simulink model "Control_model_10DOF_fin"  (R2016b)
settings: Solver=FixedStepAuto  StartTime=0.0  StopTime=10  FixedStep=0.0001  RelTol=1e-3
InitFcn:
  | Initialisation_ctr_10DOF_fin
values from neighbouring files (symbols this model uses):
  COM_Parameters = [-lpelvis/2;r2;0]    [Initialisation_ctr_10DOF_fin.m]
  DH_Parameters = [hfoot 0 ... (first row only)    [Initialisation_ctr_10DOF_fin.m]
  dTrunk = trunklbd(3)    [Initialisation_ctr_10DOF_fin.m]
  dxFootSM = dxFoot    [Initialisation_ctr_10DOF_fin.m]
  dxTrunk = 0.1    [Initialisation_ctr_10DOF_fin.m]
  Foot_Parameters = [0;-(lFoot/2-lHeel);0]    [Initialisation_ctr_10DOF_fin.m]
  HAA2HEE = [0; 0; 0.001]    [Initialisation_ctr_10DOF_fin.m]
  HEE2HFE = 0.5*[0.2; 0; 0]    [Initialisation_ctr_10DOF_fin.m]
  height_vrp = CoM_position(1)    [Initialisation_ctr_10DOF_fin.m]
  hTrunk = trunklbd(1)    [Initialisation_ctr_10DOF_fin.m]
  initial_CoM_position = R*CoM_position    [Initialisation_ctr_10DOF_fin.m]
  initial_CoM_velocity = [0;0;0]    [Initialisation_ctr_10DOF_fin.m]
  initial_left_foot = [0;0;-stance_width/2]    [Initialisation_ctr_10DOF_fin.m]
  initial_right_foot = [0;0;stance_width/2]    [Initialisation_ctr_10DOF_fin.m]
  initial_RorL = 0    [Initialisation_ctr_10DOF_fin.m]
  jointsinitial = [9;-15;6;0;0;6;-15;9]/180*pi    [Initialisation_ctr_10DOF_fin.m]
  K_DCM = 4.3*[1 0 0 ... (first row only)    [Initialisation_ctr_10DOF_fin.m]
  kD_left = mbody*[0.95 0 0 0 ... (first row only)    [Initialisation_ctr_10DOF_fin.m]
  kD_right = mbody*[0.12 0 0 0 ... (first row only)    [Initialisation_ctr_10DOF_fin.m]
  kI_left = mbody*[35 0 0 0 ... (first row only)    [Initialisation_ctr_10DOF_fin.m]
  kI_right = mbody*[38.2 0 0 0 ... (first row only)    [Initialisation_ctr_10DOF_fin.m]
  kP_left = mbody*[75 0 0 0 ... (first row only)    [Initialisation_ctr_10DOF_fin.m]
  kP_right = mbody*[5.6 0 0 0 ... (first row only)    [Initialisation_ctr_10DOF_fin.m]
  Lenght = [lShank;lThigh]    [Initialisation_ctr_10DOF_fin.m]
  lFootSM = lFoot    [Initialisation_ctr_10DOF_fin.m]
  lpelvis = wPelvis    [Initialisation_ctr_10DOF_fin.m]
  mass = mbody    (= 60)    [Initialisation_ctr_10DOF_fin.m]
  Masses = [mThigh; mShank; mTrunk]    [Initialisation_ctr_10DOF_fin.m]
  nb_step = 4    [Initialisation_ctr_10DOF_fin.m]
  nb_step_pattern = 20    [Initialisation_ctr_10DOF_fin.m]
  Pelvis_Parameters = [-lpelvis/2;hTrunk/2;0]    [Initialisation_ctr_10DOF_fin.m]
  stance_width = lpelvis    [Initialisation_ctr_10DOF_fin.m]
  stride_lenght = 0.50    (= 0.5)    [Initialisation_ctr_10DOF_fin.m]
  T_DS = time_DS    (= 0.4)    [Initialisation_ctr_10DOF_fin.m]
  T_IT = time_DS    (= 0.4)    [Initialisation_ctr_10DOF_fin.m]
  T_SS = time_swing    (= 1.6)    [Initialisation_ctr_10DOF_fin.m]
  time_DS = (time_stance-time_swing)/2    (= 0.4)    [Initialisation_ctr_10DOF_fin.m]
  time_stance = 60/100*time_stride    (= 2.4)    [Initialisation_ctr_10DOF_fin.m]
  time_step = time_stride/2    (= 2)    [Initialisation_ctr_10DOF_fin.m]
  time_swing = 40/100*time_stride    (= 1.6)    [Initialisation_ctr_10DOF_fin.m]
  validity_angle = [-20*pi/180 20*pi/180 ... (first row only)    [Initialisation_ctr_10DOF_fin.m]
  wTrunk = trunklbd(2)    [Initialisation_ctr_10DOF_fin.m]
  x4CoM = CoM_position(1)-XR4(1)    [Initialisation_ctr_10DOF_fin.m]
undefined symbols (not defined in the file or in its folder): dsegment, hFoot, l, lFoot, omega0_x, omega0_z, rho, wPelvis, X, Xp_x, Xp_z, Y, Z
undefined symbols (not defined in the file): k_grf, lShankSM, lThighSM, mShank, mThigh
libraries: nesl_utility x247, sm_lib x215, dspindex x12, FootPlacementLibrary x8, dspsigops x4, dspswit3 x1
(part 12 of 18)

== system Control_model_10DOF_fin/Control/Single_Support/Left Swing // Right Stance/Left Swing leg control/Scope x2 ==
  Input : Inport
  Input1 : Inport  Port=2
  Demux : Demux
  Demux1 : Demux
  Scope{,1..3} (4 alike) : Scope  NumInputPorts=2
  wires:
  Input/1 -> Demux/1
  Demux/2 -> Scope1/1
  Demux/3 -> Scope2/1
  Demux/1 -> Scope3/1
  Input1/1 -> Demux1/1
  Demux1/1 -> Scope3/2
  Demux1/2 -> Scope1/2
  Demux1/3 -> Scope2/2
  Demux1/4 -> Scope/2
  Demux/4 -> Scope/1

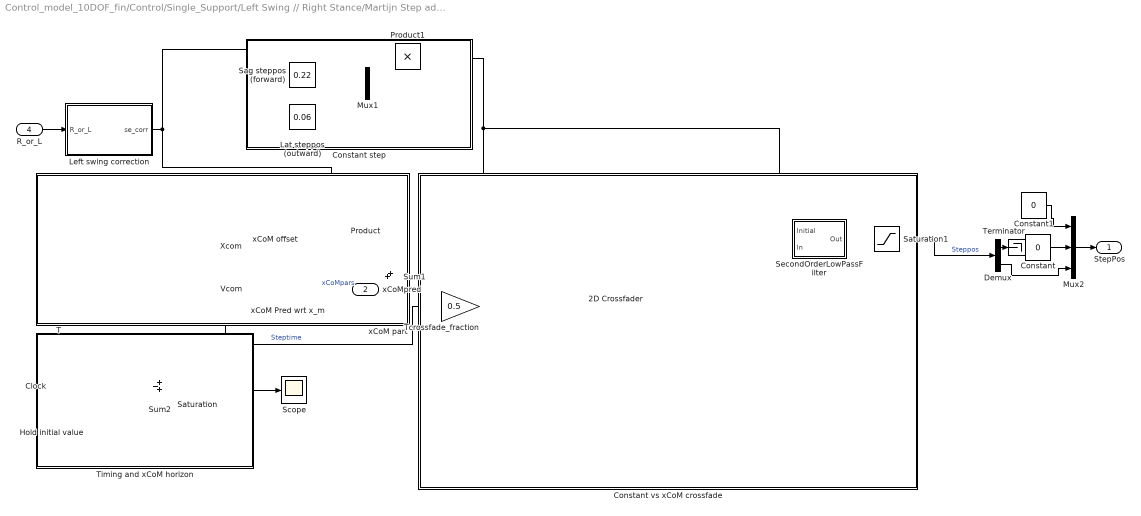
== system Control_model_10DOF_fin/Control/Single_Support/Left Swing // Right Stance/Martijn Step adjustement/xCoM pred ==
  T : Inport
  Xcom : Inport  Port=2
  Vcom : Inport  Port=3
  R_or_L : Inport  Port=4
  2D Crossfader : Subsystem
  Clock : Clock
  Constant : Constant  Value=0
  Constant step : Subsystem
  Constant vs xCoM crossfade : Subsystem
  Constant1 : Constant  Value=0
  Demux : Demux  Outputs=2
  Hold initial value : FootPlacementLibrary/Hold initial value  SystemSampleTime=-1
  Lat steppos (outward) : Constant  Value=0.06
  Left swing correction : Subsystem
  Mux1 : Mux  Inputs=2
  Mux2 : Mux  Inputs=3
  Product : Product
  Product1 : Product
  Sag steppos (forward) : Constant  Value=0.22
  Saturation : Saturate  UpperLimit=0.75  LowerLimit=0
  Saturation1 : Saturate  UpperLimit=[0.3 0.4]  LowerLimit=[-0.3 -0.4]
  Scope : Scope
  SecondOrderLowPassFilter : Subsystem  mask{w=30, z=0.7}
      mask prompts: w "Cut off omega [rad/s]"; z "Zeta"
  Sum1 : Sum  Inputs=++|
  Sum2 : Sum  Inputs=+-+
  Tcrossfade_fraction : Gain  Gain=0.5
  Terminator : Terminator
  Timing and xCoM horizon : Subsystem
  xCoM Pred wrt x_m : Subsystem
  xCoM offset : Constant  Value=[-0.120; 0.03]
  xCoM part : Subsystem
  StepPos : Outport
  xCoMpred : Outport  Port=2
  wires:
  T/1 -> Sum2/1, Tcrossfade_fraction/1  "Steptime"
  Clock/1 -> Sum2/2, Hold initial value/1
  Sum2/1 -> Saturation/1
  Hold initial value/1 -> Sum2/3
  Product/1 -> Sum1/1
  Mux1/1 -> Product1/2
  Sag steppos (forward)/1 -> Mux1/1
  Lat steppos (outward)/1 -> Mux1/2
  Left swing correction/1(se_corr) -> Product1/1, Product/1
  xCoM Pred wrt x_m/1(xCoMpred) -> Sum1/2
  Sum1/1 -> 2D Crossfader/2(xCoM)
  Tcrossfade_fraction/1 -> 2D Crossfader/3(Tcrossfade)
  Saturation/1 -> Scope/1, xCoM Pred wrt x_m/3(trem)
  Product1/1 -> 2D Crossfader/1(ConstStepPos), SecondOrderLowPassFilter/1(Initial)
  2D Crossfader/1(xCoM_crossfaded) -> SecondOrderLowPassFilter/2(In)
  xCoM offset/1 -> Product/2
  Saturation1/1 -> Demux/1  "Steppos"
  SecondOrderLowPassFilter/1(Out) -> Saturation1/1
  Vcom/1 -> xCoM Pred wrt x_m/2(v)
  Xcom/1 -> xCoM Pred wrt x_m/1(x)
  R_or_L/1 -> Left swing correction/1(R_or_L)
  Mux2/1 -> StepPos/1
  Constant/1 -> Mux2/2
  Demux/2 -> Mux2/3
  Constant1/1 -> Mux2/1
  xCoM Pred wrt x_m/2(xCoM pars) -> xCoMpred/1  "xCoMpars"
  Demux/1 -> Terminator/1

== system Control_model_10DOF_fin/Control/Single_Support/Left Swing // Right Stance/Stance leg position_initial/PID right ==
  error : Inport  PortDimensions=4
  velocity : Inport  Port=2
  Integrator : Integrator
  Product : Product  Multiplication=Matrix(*)
  Product2 : Product  Multiplication=Matrix(*)
  Product3 : Product  Multiplication=Matrix(*)
  Sum : Sum  Inputs=++-
  kD : Constant  Value=kD_right
  kI : Constant  Value=kI_right
  kP : Constant  Value=kP_right
  torques_des : Outport  PortDimensions=4  InitialOutput=0
  wires:
  Sum/1 -> torques_des/1
  Product/1 -> Sum/1
  error/1 -> Product2/2, Product/2
  kP/1 -> Product/1
  Integrator/1 -> Sum/2
  Product2/1 -> Integrator/1
  kI/1 -> Product2/1
  kD/1 -> Product3/1
  velocity/1 -> Product3/2
  Product3/1 -> Sum/3

== system Control_model_10DOF_fin/Control/Single_Support/Left Swing // Right Stance/Stance leg position_initial/Scope x2 ==
  Input : Inport
  Input1 : Inport  Port=2
  Demux : Demux
  Demux1 : Demux
  Scope{,1..3} (4 alike) : Scope  NumInputPorts=2
  wires:
  Input/1 -> Demux/1
  Demux/2 -> Scope1/1
  Demux/3 -> Scope2/1
  Demux/1 -> Scope3/1
  Input1/1 -> Demux1/1
  Demux1/1 -> Scope3/2
  Demux1/2 -> Scope1/2
  Demux1/3 -> Scope2/2
  Demux1/4 -> Scope/2
  Demux/4 -> Scope/1

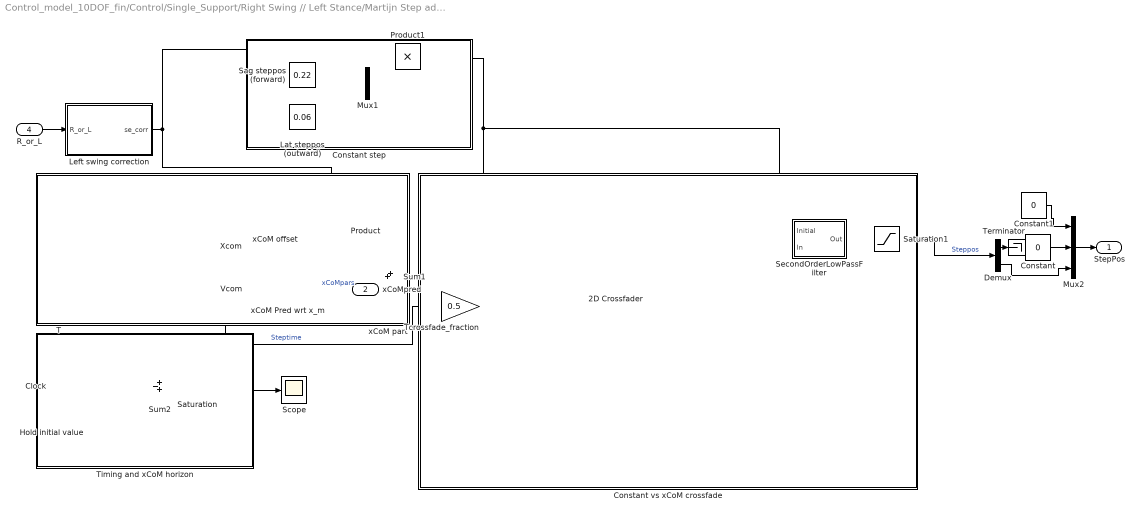
== system Control_model_10DOF_fin/Control/Single_Support/Right Swing // Left Stance/Martijn Step adjustement/xCoM pred ==
  T : Inport
  Xcom : Inport  Port=2
  Vcom : Inport  Port=3
  R_or_L : Inport  Port=4
  2D Crossfader : Subsystem
  Clock : Clock
  Constant : Constant  Value=0
  Constant step : Subsystem
  Constant vs xCoM crossfade : Subsystem
  Constant1 : Constant  Value=0
  Demux : Demux  Outputs=2
  Hold initial value : FootPlacementLibrary/Hold initial value  SystemSampleTime=-1
  Lat steppos (outward) : Constant  Value=0.06
  Left swing correction : Subsystem
  Mux1 : Mux  Inputs=2
  Mux2 : Mux  Inputs=3
  Product : Product
  Product1 : Product
  Sag steppos (forward) : Constant  Value=0.22
  Saturation : Saturate  UpperLimit=0.75  LowerLimit=0
  Saturation1 : Saturate  UpperLimit=[0.3 0.4]  LowerLimit=[-0.3 -0.4]
  Scope : Scope
  SecondOrderLowPassFilter : Subsystem  mask{w=30, z=0.7}
      mask prompts: w "Cut off omega [rad/s]"; z "Zeta"
  Sum1 : Sum  Inputs=++|
  Sum2 : Sum  Inputs=+-+
  Tcrossfade_fraction : Gain  Gain=0.5
  Terminator : Terminator
  Timing and xCoM horizon : Subsystem
  xCoM Pred wrt x_m : Subsystem
  xCoM offset : Constant  Value=[-0.120; 0.03]
  xCoM part : Subsystem
  StepPos : Outport
  xCoMpred : Outport  Port=2
  wires:
  T/1 -> Sum2/1, Tcrossfade_fraction/1  "Steptime"
  Clock/1 -> Sum2/2, Hold initial value/1
  Sum2/1 -> Saturation/1
  Hold initial value/1 -> Sum2/3
  Product/1 -> Sum1/1
  Mux1/1 -> Product1/2
  Sag steppos (forward)/1 -> Mux1/1
  Lat steppos (outward)/1 -> Mux1/2
  Left swing correction/1(se_corr) -> Product1/1, Product/1
  xCoM Pred wrt x_m/1(xCoMpred) -> Sum1/2
  Sum1/1 -> 2D Crossfader/2(xCoM)
  Tcrossfade_fraction/1 -> 2D Crossfader/3(Tcrossfade)
  Saturation/1 -> Scope/1, xCoM Pred wrt x_m/3(trem)
  Product1/1 -> 2D Crossfader/1(ConstStepPos), SecondOrderLowPassFilter/1(Initial)
  2D Crossfader/1(xCoM_crossfaded) -> SecondOrderLowPassFilter/2(In)
  xCoM offset/1 -> Product/2
  Saturation1/1 -> Demux/1  "Steppos"
  SecondOrderLowPassFilter/1(Out) -> Saturation1/1
  Vcom/1 -> xCoM Pred wrt x_m/2(v)
  Xcom/1 -> xCoM Pred wrt x_m/1(x)
  R_or_L/1 -> Left swing correction/1(R_or_L)
  Mux2/1 -> StepPos/1
  Constant/1 -> Mux2/2
  Demux/2 -> Mux2/3
  Constant1/1 -> Mux2/1
  xCoM Pred wrt x_m/2(xCoM pars) -> xCoMpred/1  "xCoMpars"
  Demux/1 -> Terminator/1

== system Control_model_10DOF_fin/Control/Single_Support/Right Swing // Left Stance/Right Swing leg control/PID right ==
  error : Inport  PortDimensions=4
  velocity : Inport  Port=2
  Integrator : Integrator
  Product : Product  Multiplication=Matrix(*)
  Product2 : Product  Multiplication=Matrix(*)
  Product3 : Product  Multiplication=Matrix(*)
  Sum : Sum  Inputs=++-
  kD : Constant  Value=kD_right
  kI : Constant  Value=kI_right
  kP : Constant  Value=kP_right
  torques_des : Outport  PortDimensions=4  InitialOutput=0
  wires:
  Sum/1 -> torques_des/1
  Product/1 -> Sum/1
  error/1 -> Product2/2, Product/2
  kP/1 -> Product/1
  Integrator/1 -> Sum/2
  Product2/1 -> Integrator/1
  kI/1 -> Product2/1
  kD/1 -> Product3/1
  velocity/1 -> Product3/2
  Product3/1 -> Sum/3

== system Control_model_10DOF_fin/Control/Single_Support/Right Swing // Left Stance/Right Swing leg control/Scope x2 ==
  Input : Inport
  Input1 : Inport  Port=2
  Demux : Demux
  Demux1 : Demux
  Gain : Gain  Gain=180/pi
  Gain1 : Gain  Gain=180/pi
  Scope{,1..3} (4 alike) : Scope  NumInputPorts=2
  wires:
  Input/1 -> Gain/1
  Demux/2 -> Scope1/1
  Demux/3 -> Scope2/1
  Demux/1 -> Scope3/1
  Input1/1 -> Gain1/1
  Demux1/1 -> Scope3/2
  Demux1/2 -> Scope1/2
  Demux1/3 -> Scope2/2
  Demux1/4 -> Scope/2
  Demux/4 -> Scope/1
  Gain/1 -> Demux/1
  Gain1/1 -> Demux1/1

== system Control_model_10DOF_fin/Control/Single_Support/Right Swing // Left Stance/Stance leg position_initial1/PID left ==
  error : Inport  PortDimensions=4
  velocity : Inport  Port=2
  Integrator : Integrator
  Product : Product  Multiplication=Matrix(*)
  Product2 : Product  Multiplication=Matrix(*)
  Product3 : Product  Multiplication=Matrix(*)
  Sum : Sum  Inputs=++-
  kD : Constant  Value=kD_left
  kI : Constant  Value=kI_left
  kP : Constant  Value=kP_left
  torques_des : Outport  PortDimensions=4  InitialOutput=0
  wires:
  Sum/1 -> torques_des/1
  Product/1 -> Sum/1
  error/1 -> Product2/2, Product/2
  kP/1 -> Product/1
  Integrator/1 -> Sum/2
  Product2/1 -> Integrator/1
  kI/1 -> Product2/1
  kD/1 -> Product3/1
  velocity/1 -> Product3/2
  Product3/1 -> Sum/3

== system Control_model_10DOF_fin/Trajectory generator/Enabled and Triggered Subsystem 1/Feet Pattern generator/initial position/initial position ==
  Action Port : ActionPort  ActionType=then
  Constant : Constant  Value=initial_right_foot
  Constant1 : Constant  Value=initial_left_foot
  initial_swing_foot : Outport
  initial_stance_foot : Outport  Port=2
  wires:
  Constant/1 -> initial_swing_foot/1
  Constant1/1 -> initial_stance_foot/1

== system Control_model_10DOF_fin/Trajectory generator/Enabled and Triggered Subsystem 1/Feet Pattern generator/initial position/initial position1 ==
  Action Port : ActionPort  ActionType=else
  Constant : Constant  Value=initial_left_foot
  Constant1 : Constant  Value=initial_right_foot
  initial_swing_foot : Outport
  initial_stance_foot : Outport  Port=2
  wires:
  Constant/1 -> initial_swing_foot/1
  Constant1/1 -> initial_stance_foot/1

== system Control_model_10DOF_fin/Trajectory generator/Hip trajectory2/SS/Subsystem2/Subsystem ==
  time_Hip : Inport
  Action Port : ActionPort  InitializeStates=reset  ActionType=else
  Hip trajectory : MATLAB Function  TreatAsAtomicUnit=on
  hip_trajectory : Outport
  wires:
  Hip trajectory/1(hip_angle_des) -> hip_trajectory/1
  time_Hip/1 -> Hip trajectory/1(current_time)

== system Control_model_10DOF_fin/Trajectory generator/Hip trajectory2/SS/Subsystem2/Subsystem1 ==
  Action Port : ActionPort  InitializeStates=reset  ActionType=then
  Constant : Constant  Value=-3.3*pi/180
  hip_trajectory : Outport
  wires:
  Constant/1 -> hip_trajectory/1

== system Control_model_10DOF_fin/Trajectory generator/knee trajectory/SS/Left swing /knee trajectory ==
  current_time : Inport  OutDataTypeStr=double  Unit=s  PortDimensions=1
  knee_angle_ini : Inport  Port=2
  Action Port : ActionPort  ActionType=then
  Swing leg trajectory1 : MATLAB Function  TreatAsAtomicUnit=on
  knee_angle_des : Outport
  knee_angle_des2 : Outport  Port=2
  wires:
  current_time/1 -> Swing leg trajectory1/1(current_time)
  Swing leg trajectory1/1(knee_angle_des) -> knee_angle_des2/1, knee_angle_des/1
  knee_angle_ini/1 -> Swing leg trajectory1/2(knee_angle_ini)

== system Control_model_10DOF_fin/Trajectory generator/knee trajectory/SS/Left swing /knee trajectory1 ==
  current_time : Inport  OutDataTypeStr=double  Unit=m  PortDimensions=1
  knee_angle_ini : Inport  Port=2
  Action Port : ActionPort  ActionType=else
  Swing leg trajectory1 : MATLAB Function  TreatAsAtomicUnit=on
  knee_angle_des : Outport
  wires:
  current_time/1 -> Swing leg trajectory1/1(current_time)
  Swing leg trajectory1/1(knee_angle_des) -> knee_angle_des/1
  knee_angle_ini/1 -> Swing leg trajectory1/2(knee_angle_ini)

== system Control_model_10DOF_fin/Trajectory generator/knee trajectory/SS/Right swing/knee trajectory ==
  current_time : Inport  OutDataTypeStr=double  Unit=s  PortDimensions=1
  knee_angle_ini : Inport  Port=2
  Action Port : ActionPort  ActionType=then
  Swing leg trajectory1 : MATLAB Function  TreatAsAtomicUnit=on
  knee_angle_des : Outport
  knee_angle_des2 : Outport  Port=2
  wires:
  current_time/1 -> Swing leg trajectory1/1(current_time)
  Swing leg trajectory1/1(knee_angle_des) -> knee_angle_des2/1, knee_angle_des/1
  knee_angle_ini/1 -> Swing leg trajectory1/2(knee_angle_ini)

== system Control_model_10DOF_fin/Trajectory generator/knee trajectory/SS/Right swing/knee trajectory1 ==
  current_time : Inport  OutDataTypeStr=double  Unit=m  PortDimensions=1
  knee_angle_ini : Inport  Port=2
  Action Port : ActionPort  ActionType=else
  Swing leg trajectory1 : MATLAB Function  TreatAsAtomicUnit=on
  knee_angle_des : Outport
  wires:
  current_time/1 -> Swing leg trajectory1/1(current_time)
  Swing leg trajectory1/1(knee_angle_des) -> knee_angle_des/1
  knee_angle_ini/1 -> Swing leg trajectory1/2(knee_angle_ini)

== system Control_model_10DOF_fin/Control/Finish_Swing_Phase/Left Swing // Right Stance/Martijn Step adjustement/xCoM pred/2D Crossfader ==
  ConstStepPos : Inport
  xCoM : Inport  Port=2
  Tcrossfade : Inport  Port=3
  1D 2Node Cubic Spline : FootPlacementLibrary/1D 2Node Cubic Spline  extrapol=Maintain boundary value
  Constant : Constant  Value=0
  Constant4 : Constant
  Max xCoM share : Constant
  MergeGain : Gain
  Product2 : Product  RndMeth=Zero
  Product3 : Product  RndMeth=Zero
  Sum : Sum  Inputs=|-+
  Sum3 : Sum
  Terminator : Terminator
  xCoM_crossfaded : Outport
  wires:
  Sum3/1 -> MergeGain/1
  Tcrossfade/1 -> 1D 2Node Cubic Spline/3
  Product3/1 -> Sum3/2
  Product2/1 -> Sum3/1
  Sum/1 -> Product3/1
  Constant4/1 -> Sum/2
  1D 2Node Cubic Spline/1 -> Sum/1, Product2/2
  Max xCoM share/1 -> 1D 2Node Cubic Spline/4
  ConstStepPos/1 -> Product3/2
  xCoM/1 -> Product2/1
  MergeGain/1 -> xCoM_crossfaded/1
  1D 2Node Cubic Spline/2 -> Terminator/1
  Constant/1 -> 1D 2Node Cubic Spline/6, 1D 2Node Cubic Spline/5, 1D 2Node Cubic Spline/2, 1D 2Node Cubic Spline/1

== system Control_model_10DOF_fin/Control/Finish_Swing_Phase/Left Swing // Right Stance/Martijn Step adjustement/xCoM pred/Constant step ==

== system Control_model_10DOF_fin/Control/Finish_Swing_Phase/Left Swing // Right Stance/Martijn Step adjustement/xCoM pred/Constant vs xCoM crossfade ==

== system Control_model_10DOF_fin/Control/Finish_Swing_Phase/Left Swing // Right Stance/Martijn Step adjustement/xCoM pred/Left swing correction ==
  R_or_L : Inport
  If Right stance / Left swing : If  IfExpression=u1 ==1
  Left Swing : Subsystem  TreatAsAtomicUnit=on
  Merge : Merge
  Right Swing : Subsystem  TreatAsAtomicUnit=on
  se_corr : Outport
  wires:
  R_or_L/1 -> If Right stance / Left swing/1
  If Right stance / Left swing/1 -> Right Swing/Action
  If Right stance / Left swing/2 -> Left Swing/Action
  Merge/1 -> se_corr/1
  Right Swing/1(se_corr) -> Merge/1
  Left Swing/1(se_corr) -> Merge/2

== system Control_model_10DOF_fin/Control/Finish_Swing_Phase/Left Swing // Right Stance/Martijn Step adjustement/xCoM pred/SecondOrderLowPassFilter ==
  note: This is an implementation of a
      | second order low pass filter with
      | settable zeta and omega.
      | It works for scalars as well as vectors.
      |
      | You can monitor the output from Python
      | by monitoring OutputValue.s[0,:]
  Initial : Inport
  In : Inport  Port=2
  Integrator : Integrator
  OutputValue : Integrator  InitialConditionSource=external  InitialCondition=[0.1 0.0]
  Product1 : Product  RndMeth=Zero
  Product2 : Product  RndMeth=Zero
  Sum : Sum  Inputs=|+-
  Sum1 : Sum  Inputs=|+-
  omega : Constant  Value=w
  omega_sq : Math  Operator=square  SaturateOnIntegerOverflow=on
  two : Constant  Value=2
  zeta : Constant  Value=z
  zeta_omega_2 : Product  Inputs=3  RndMeth=Zero
  Out : Outport
  wires:
  OutputValue/1 -> Out/1, Sum/2
  Sum1/1 -> Integrator/1
  In/1 -> Sum/1
  Integrator/1 -> Product2/1, OutputValue/1
  Sum/1 -> Product1/1
  omega/1 -> zeta_omega_2/3, omega_sq/1
  two/1 -> zeta_omega_2/1
  zeta/1 -> zeta_omega_2/2
  omega_sq/1 -> Product1/2
  Product1/1 -> Sum1/1
  zeta_omega_2/1 -> Product2/2
  Product2/1 -> Sum1/2
  Initial/1 -> OutputValue/2

== system Control_model_10DOF_fin/Control/Finish_Swing_Phase/Left Swing // Right Stance/Martijn Step adjustement/xCoM pred/Timing and xCoM horizon ==

== system Control_model_10DOF_fin/Control/Finish_Swing_Phase/Left Swing // Right Stance/Martijn Step adjustement/xCoM pred/xCoM Pred wrt x_m ==
  x : Inport
  v : Inport  Port=2
  trem : Inport  Port=3
  Constant1 : Constant  Value=Xp_x
  Constant2 : Constant  Value=omega0_z
  Constant3 : Constant  Value=Xp_z
  Demux : Demux  Outputs=3
  Demux1 : Demux  Outputs=3
  Gain : Gain
  Gain1 : Gain
  Mux : Mux  Inputs=2
  Mux1 : Mux  Inputs=5
  Terminator : Terminator
  Terminator1 : Terminator
  one2 : Constant  Value=omega0_x
  xCoM Pred Rel : Subsystem
  xCoM Pred Rel1 : Subsystem
  xCoMpred : Outport
  xCoM pars : Outport  Port=2
  wires:
  x/1 -> Demux/1
  trem/1 -> xCoM Pred Rel1/5(T-t0), Mux1/5, xCoM Pred Rel/5(T-t0)
  v/1 -> Demux1/1
  xCoM Pred Rel/1(xCoM Pred) -> Mux/1
  xCoM Pred Rel1/1(xCoM Pred) -> Mux/2
  Mux/1 -> xCoMpred/1
  Constant1/1 -> Mux1/2, xCoM Pred Rel/4(Xp)
  Constant3/1 -> Mux1/4, xCoM Pred Rel1/4(Xp)
  Gain/1 -> Mux1/1, xCoM Pred Rel/3(w0)
  Gain1/1 -> Mux1/3, xCoM Pred Rel1/3(w0)
  Mux1/1 -> xCoM pars/1
  one2/1 -> Gain/1
  Constant2/1 -> Gain1/1
  Demux/3 -> xCoM Pred Rel1/1(x)
  Demux1/3 -> xCoM Pred Rel1/2(v)
  Demux/1 -> xCoM Pred Rel/1(x)
  Demux1/1 -> xCoM Pred Rel/2(v)
  Demux/2 -> Terminator/1
  Demux1/2 -> Terminator1/1

== system Control_model_10DOF_fin/Control/Finish_Swing_Phase/Left Swing // Right Stance/Martijn Step adjustement/xCoM pred/xCoM part ==

== system Control_model_10DOF_fin/Control/Finish_Swing_Phase/Right Swing // Left Stance1/Martijn Step adjustement/xCoM pred/2D Crossfader ==
  ConstStepPos : Inport
  xCoM : Inport  Port=2
  Tcrossfade : Inport  Port=3
  1D 2Node Cubic Spline : FootPlacementLibrary/1D 2Node Cubic Spline  extrapol=Maintain boundary value
  Constant : Constant  Value=0
  Constant4 : Constant
  Max xCoM share : Constant
  MergeGain : Gain
  Product2 : Product  RndMeth=Zero
  Product3 : Product  RndMeth=Zero
  Sum : Sum  Inputs=|-+
  Sum3 : Sum
  Terminator : Terminator
  xCoM_crossfaded : Outport
  wires:
  Sum3/1 -> MergeGain/1
  Tcrossfade/1 -> 1D 2Node Cubic Spline/3
  Product3/1 -> Sum3/2
  Product2/1 -> Sum3/1
  Sum/1 -> Product3/1
  Constant4/1 -> Sum/2
  1D 2Node Cubic Spline/1 -> Sum/1, Product2/2
  Max xCoM share/1 -> 1D 2Node Cubic Spline/4
  ConstStepPos/1 -> Product3/2
  xCoM/1 -> Product2/1
  MergeGain/1 -> xCoM_crossfaded/1
  1D 2Node Cubic Spline/2 -> Terminator/1
  Constant/1 -> 1D 2Node Cubic Spline/6, 1D 2Node Cubic Spline/5, 1D 2Node Cubic Spline/2, 1D 2Node Cubic Spline/1

== system Control_model_10DOF_fin/Control/Finish_Swing_Phase/Right Swing // Left Stance1/Martijn Step adjustement/xCoM pred/Constant step ==

== system Control_model_10DOF_fin/Control/Finish_Swing_Phase/Right Swing // Left Stance1/Martijn Step adjustement/xCoM pred/Constant vs xCoM crossfade ==

== system Control_model_10DOF_fin/Control/Finish_Swing_Phase/Right Swing // Left Stance1/Martijn Step adjustement/xCoM pred/Left swing correction ==
  R_or_L : Inport
  If Right stance / Left swing : If  IfExpression=u1 ==1
  Left Swing : Subsystem  TreatAsAtomicUnit=on
  Merge : Merge
  Right Swing : Subsystem  TreatAsAtomicUnit=on
  se_corr : Outport
  wires:
  R_or_L/1 -> If Right stance / Left swing/1
  If Right stance / Left swing/1 -> Right Swing/Action
  If Right stance / Left swing/2 -> Left Swing/Action
  Merge/1 -> se_corr/1
  Right Swing/1(se_corr) -> Merge/1
  Left Swing/1(se_corr) -> Merge/2

== system Control_model_10DOF_fin/Control/Finish_Swing_Phase/Right Swing // Left Stance1/Martijn Step adjustement/xCoM pred/SecondOrderLowPassFilter ==
  note: This is an implementation of a
      | second order low pass filter with
      | settable zeta and omega.
      | It works for scalars as well as vectors.
      |
      | You can monitor the output from Python
      | by monitoring OutputValue.s[0,:]
  Initial : Inport
  In : Inport  Port=2
  Integrator : Integrator
  OutputValue : Integrator  InitialConditionSource=external  InitialCondition=[0.1 0.0]
  Product1 : Product  RndMeth=Zero
  Product2 : Product  RndMeth=Zero
  Sum : Sum  Inputs=|+-
  Sum1 : Sum  Inputs=|+-
  omega : Constant  Value=w
  omega_sq : Math  Operator=square  SaturateOnIntegerOverflow=on
  two : Constant  Value=2
  zeta : Constant  Value=z
  zeta_omega_2 : Product  Inputs=3  RndMeth=Zero
  Out : Outport
  wires:
  OutputValue/1 -> Out/1, Sum/2
  Sum1/1 -> Integrator/1
  In/1 -> Sum/1
  Integrator/1 -> Product2/1, OutputValue/1
  Sum/1 -> Product1/1
  omega/1 -> zeta_omega_2/3, omega_sq/1
  two/1 -> zeta_omega_2/1
  zeta/1 -> zeta_omega_2/2
  omega_sq/1 -> Product1/2
  Product1/1 -> Sum1/1
  zeta_omega_2/1 -> Product2/2
  Product2/1 -> Sum1/2
  Initial/1 -> OutputValue/2

== system Control_model_10DOF_fin/Control/Finish_Swing_Phase/Right Swing // Left Stance1/Martijn Step adjustement/xCoM pred/Timing and xCoM horizon ==

== system Control_model_10DOF_fin/Control/Finish_Swing_Phase/Right Swing // Left Stance1/Martijn Step adjustement/xCoM pred/xCoM Pred wrt x_m ==
  x : Inport
  v : Inport  Port=2
  trem : Inport  Port=3
  Constant1 : Constant  Value=Xp_x
  Constant2 : Constant  Value=omega0_z
  Constant3 : Constant  Value=Xp_z
  Demux : Demux  Outputs=3
  Demux1 : Demux  Outputs=3
  Gain : Gain
  Gain1 : Gain
  Mux : Mux  Inputs=2
  Mux1 : Mux  Inputs=5
  Terminator : Terminator
  Terminator1 : Terminator
  one2 : Constant  Value=omega0_x
  xCoM Pred Rel : Subsystem
  xCoM Pred Rel1 : Subsystem
  xCoMpred : Outport
  xCoM pars : Outport  Port=2
  wires:
  x/1 -> Demux/1
  trem/1 -> xCoM Pred Rel1/5(T-t0), Mux1/5, xCoM Pred Rel/5(T-t0)
  v/1 -> Demux1/1
  xCoM Pred Rel/1(xCoM Pred) -> Mux/1
  xCoM Pred Rel1/1(xCoM Pred) -> Mux/2
  Mux/1 -> xCoMpred/1
  Constant1/1 -> Mux1/2, xCoM Pred Rel/4(Xp)
  Constant3/1 -> Mux1/4, xCoM Pred Rel1/4(Xp)
  Gain/1 -> Mux1/1, xCoM Pred Rel/3(w0)
  Gain1/1 -> Mux1/3, xCoM Pred Rel1/3(w0)
  Mux1/1 -> xCoM pars/1
  one2/1 -> Gain/1
  Constant2/1 -> Gain1/1
  Demux/3 -> xCoM Pred Rel1/1(x)
  Demux1/3 -> xCoM Pred Rel1/2(v)
  Demux/1 -> xCoM Pred Rel/1(x)
  Demux1/1 -> xCoM Pred Rel/2(v)
  Demux/2 -> Terminator/1
  Demux1/2 -> Terminator1/1

== system Control_model_10DOF_fin/Control/Finish_Swing_Phase/Right Swing // Left Stance1/Martijn Step adjustement/xCoM pred/xCoM part ==

== system Control_model_10DOF_fin/Control/Single_Support/Left Swing // Right Stance/Martijn Step adjustement/xCoM pred/2D Crossfader ==
  ConstStepPos : Inport
  xCoM : Inport  Port=2
  Tcrossfade : Inport  Port=3
  1D 2Node Cubic Spline : FootPlacementLibrary/1D 2Node Cubic Spline  extrapol=Maintain boundary value
  Constant : Constant  Value=0
  Constant4 : Constant
  Max xCoM share : Constant
  MergeGain : Gain
  Product2 : Product  RndMeth=Zero
  Product3 : Product  RndMeth=Zero
  Sum : Sum  Inputs=|-+
  Sum3 : Sum
  Terminator : Terminator
  xCoM_crossfaded : Outport
  wires:
  Sum3/1 -> MergeGain/1
  Tcrossfade/1 -> 1D 2Node Cubic Spline/3
  Product3/1 -> Sum3/2
  Product2/1 -> Sum3/1
  Sum/1 -> Product3/1
  Constant4/1 -> Sum/2
  1D 2Node Cubic Spline/1 -> Sum/1, Product2/2
  Max xCoM share/1 -> 1D 2Node Cubic Spline/4
  ConstStepPos/1 -> Product3/2
  xCoM/1 -> Product2/1
  MergeGain/1 -> xCoM_crossfaded/1
  1D 2Node Cubic Spline/2 -> Terminator/1
  Constant/1 -> 1D 2Node Cubic Spline/6, 1D 2Node Cubic Spline/5, 1D 2Node Cubic Spline/2, 1D 2Node Cubic Spline/1

== system Control_model_10DOF_fin/Control/Single_Support/Left Swing // Right Stance/Martijn Step adjustement/xCoM pred/Constant step ==

== system Control_model_10DOF_fin/Control/Single_Support/Left Swing // Right Stance/Martijn Step adjustement/xCoM pred/Constant vs xCoM crossfade ==

== system Control_model_10DOF_fin/Control/Single_Support/Left Swing // Right Stance/Martijn Step adjustement/xCoM pred/Left swing correction ==
  R_or_L : Inport
  If Right stance / Left swing : If  IfExpression=u1 ==1
  Left Swing : Subsystem  TreatAsAtomicUnit=on
  Merge : Merge
  Right Swing : Subsystem  TreatAsAtomicUnit=on
  se_corr : Outport
  wires:
  R_or_L/1 -> If Right stance / Left swing/1
  If Right stance / Left swing/1 -> Right Swing/Action
  If Right stance / Left swing/2 -> Left Swing/Action
  Merge/1 -> se_corr/1
  Right Swing/1(se_corr) -> Merge/1
  Left Swing/1(se_corr) -> Merge/2

== system Control_model_10DOF_fin/Control/Single_Support/Left Swing // Right Stance/Martijn Step adjustement/xCoM pred/SecondOrderLowPassFilter ==
  note: This is an implementation of a
      | second order low pass filter with
      | settable zeta and omega.
      | It works for scalars as well as vectors.
      |
      | You can monitor the output from Python
      | by monitoring OutputValue.s[0,:]
  Initial : Inport
  In : Inport  Port=2
  Integrator : Integrator
  OutputValue : Integrator  InitialConditionSource=external  InitialCondition=[0.1 0.0]
  Product1 : Product  RndMeth=Zero
  Product2 : Product  RndMeth=Zero
  Sum : Sum  Inputs=|+-
  Sum1 : Sum  Inputs=|+-
  omega : Constant  Value=w
  omega_sq : Math  Operator=square  SaturateOnIntegerOverflow=on
  two : Constant  Value=2
  zeta : Constant  Value=z
  zeta_omega_2 : Product  Inputs=3  RndMeth=Zero
  Out : Outport
  wires:
  OutputValue/1 -> Out/1, Sum/2
  Sum1/1 -> Integrator/1
  In/1 -> Sum/1
  Integrator/1 -> Product2/1, OutputValue/1
  Sum/1 -> Product1/1
  omega/1 -> zeta_omega_2/3, omega_sq/1
  two/1 -> zeta_omega_2/1
  zeta/1 -> zeta_omega_2/2
  omega_sq/1 -> Product1/2
  Product1/1 -> Sum1/1
  zeta_omega_2/1 -> Product2/2
  Product2/1 -> Sum1/2
  Initial/1 -> OutputValue/2

== system Control_model_10DOF_fin/Control/Single_Support/Left Swing // Right Stance/Martijn Step adjustement/xCoM pred/Timing and xCoM horizon ==

== system Control_model_10DOF_fin/Control/Single_Support/Left Swing // Right Stance/Martijn Step adjustement/xCoM pred/xCoM Pred wrt x_m ==
  x : Inport
  v : Inport  Port=2
  trem : Inport  Port=3
  Constant1 : Constant  Value=Xp_x
  Constant2 : Constant  Value=omega0_z
  Constant3 : Constant  Value=Xp_z
  Demux : Demux  Outputs=3
  Demux1 : Demux  Outputs=3
  Gain : Gain
  Gain1 : Gain
  Mux : Mux  Inputs=2
  Mux1 : Mux  Inputs=5
  Terminator : Terminator
  Terminator1 : Terminator
  one2 : Constant  Value=omega0_x
  xCoM Pred Rel : Subsystem
  xCoM Pred Rel1 : Subsystem
  xCoMpred : Outport
  xCoM pars : Outport  Port=2
  wires:
  x/1 -> Demux/1
  trem/1 -> xCoM Pred Rel1/5(T-t0), Mux1/5, xCoM Pred Rel/5(T-t0)
  v/1 -> Demux1/1
  xCoM Pred Rel/1(xCoM Pred) -> Mux/1
  xCoM Pred Rel1/1(xCoM Pred) -> Mux/2
  Mux/1 -> xCoMpred/1
  Constant1/1 -> Mux1/2, xCoM Pred Rel/4(Xp)
  Constant3/1 -> Mux1/4, xCoM Pred Rel1/4(Xp)
  Gain/1 -> Mux1/1, xCoM Pred Rel/3(w0)
  Gain1/1 -> Mux1/3, xCoM Pred Rel1/3(w0)
  Mux1/1 -> xCoM pars/1
  one2/1 -> Gain/1
  Constant2/1 -> Gain1/1
  Demux/3 -> xCoM Pred Rel1/1(x)
  Demux1/3 -> xCoM Pred Rel1/2(v)
  Demux/1 -> xCoM Pred Rel/1(x)
  Demux1/1 -> xCoM Pred Rel/2(v)
  Demux/2 -> Terminator/1
  Demux1/2 -> Terminator1/1

== system Control_model_10DOF_fin/Control/Single_Support/Left Swing // Right Stance/Martijn Step adjustement/xCoM pred/xCoM part ==

== system Control_model_10DOF_fin/Control/Single_Support/Right Swing // Left Stance/Martijn Step adjustement/xCoM pred/2D Crossfader ==
  ConstStepPos : Inport
  xCoM : Inport  Port=2
  Tcrossfade : Inport  Port=3
  1D 2Node Cubic Spline : FootPlacementLibrary/1D 2Node Cubic Spline  extrapol=Maintain boundary value
  Constant : Constant  Value=0
  Constant4 : Constant
  Max xCoM share : Constant
  MergeGain : Gain
  Product2 : Product  RndMeth=Zero
  Product3 : Product  RndMeth=Zero
  Sum : Sum  Inputs=|-+
  Sum3 : Sum
  Terminator : Terminator
  xCoM_crossfaded : Outport
  wires:
  Sum3/1 -> MergeGain/1
  Tcrossfade/1 -> 1D 2Node Cubic Spline/3
  Product3/1 -> Sum3/2
  Product2/1 -> Sum3/1
  Sum/1 -> Product3/1
  Constant4/1 -> Sum/2
  1D 2Node Cubic Spline/1 -> Sum/1, Product2/2
  Max xCoM share/1 -> 1D 2Node Cubic Spline/4
  ConstStepPos/1 -> Product3/2
  xCoM/1 -> Product2/1
  MergeGain/1 -> xCoM_crossfaded/1
  1D 2Node Cubic Spline/2 -> Terminator/1
  Constant/1 -> 1D 2Node Cubic Spline/6, 1D 2Node Cubic Spline/5, 1D 2Node Cubic Spline/2, 1D 2Node Cubic Spline/1

== system Control_model_10DOF_fin/Control/Single_Support/Right Swing // Left Stance/Martijn Step adjustement/xCoM pred/Constant step ==

== system Control_model_10DOF_fin/Control/Single_Support/Right Swing // Left Stance/Martijn Step adjustement/xCoM pred/Constant vs xCoM crossfade ==

== system Control_model_10DOF_fin/Control/Single_Support/Right Swing // Left Stance/Martijn Step adjustement/xCoM pred/Left swing correction ==
  R_or_L : Inport
  If Right stance / Left swing : If  IfExpression=u1 ==1
  Left Swing : Subsystem  TreatAsAtomicUnit=on
  Merge : Merge
  Right Swing : Subsystem  TreatAsAtomicUnit=on
  se_corr : Outport
  wires:
  R_or_L/1 -> If Right stance / Left swing/1
  If Right stance / Left swing/1 -> Right Swing/Action
  If Right stance / Left swing/2 -> Left Swing/Action
  Merge/1 -> se_corr/1
  Right Swing/1(se_corr) -> Merge/1
  Left Swing/1(se_corr) -> Merge/2

== system Control_model_10DOF_fin/Control/Single_Support/Right Swing // Left Stance/Martijn Step adjustement/xCoM pred/SecondOrderLowPassFilter ==
  note: This is an implementation of a
      | second order low pass filter with
      | settable zeta and omega.
      | It works for scalars as well as vectors.
      |
      | You can monitor the output from Python
      | by monitoring OutputValue.s[0,:]
  Initial : Inport
  In : Inport  Port=2
  Integrator : Integrator
  OutputValue : Integrator  InitialConditionSource=external  InitialCondition=[0.1 0.0]
  Product1 : Product  RndMeth=Zero
  Product2 : Product  RndMeth=Zero
  Sum : Sum  Inputs=|+-
  Sum1 : Sum  Inputs=|+-
  omega : Constant  Value=w
  omega_sq : Math  Operator=square  SaturateOnIntegerOverflow=on
  two : Constant  Value=2
  zeta : Constant  Value=z
  zeta_omega_2 : Product  Inputs=3  RndMeth=Zero
  Out : Outport
  wires:
  OutputValue/1 -> Out/1, Sum/2
  Sum1/1 -> Integrator/1
  In/1 -> Sum/1
  Integrator/1 -> Product2/1, OutputValue/1
  Sum/1 -> Product1/1
  omega/1 -> zeta_omega_2/3, omega_sq/1
  two/1 -> zeta_omega_2/1
  zeta/1 -> zeta_omega_2/2
  omega_sq/1 -> Product1/2
  Product1/1 -> Sum1/1
  zeta_omega_2/1 -> Product2/2
  Product2/1 -> Sum1/2
  Initial/1 -> OutputValue/2

== system Control_model_10DOF_fin/Control/Single_Support/Right Swing // Left Stance/Martijn Step adjustement/xCoM pred/Timing and xCoM horizon ==

== system Control_model_10DOF_fin/Control/Single_Support/Right Swing // Left Stance/Martijn Step adjustement/xCoM pred/xCoM Pred wrt x_m ==
  x : Inport
  v : Inport  Port=2
  trem : Inport  Port=3
  Constant1 : Constant  Value=Xp_x
  Constant2 : Constant  Value=omega0_z
  Constant3 : Constant  Value=Xp_z
  Demux : Demux  Outputs=3
  Demux1 : Demux  Outputs=3
  Gain : Gain
  Gain1 : Gain
  Mux : Mux  Inputs=2
  Mux1 : Mux  Inputs=5
  Terminator : Terminator
  Terminator1 : Terminator
  one2 : Constant  Value=omega0_x
  xCoM Pred Rel : Subsystem
  xCoM Pred Rel1 : Subsystem
  xCoMpred : Outport
  xCoM pars : Outport  Port=2
  wires:
  x/1 -> Demux/1
  trem/1 -> xCoM Pred Rel1/5(T-t0), Mux1/5, xCoM Pred Rel/5(T-t0)
  v/1 -> Demux1/1
  xCoM Pred Rel/1(xCoM Pred) -> Mux/1
  xCoM Pred Rel1/1(xCoM Pred) -> Mux/2
  Mux/1 -> xCoMpred/1
  Constant1/1 -> Mux1/2, xCoM Pred Rel/4(Xp)
  Constant3/1 -> Mux1/4, xCoM Pred Rel1/4(Xp)
  Gain/1 -> Mux1/1, xCoM Pred Rel/3(w0)
  Gain1/1 -> Mux1/3, xCoM Pred Rel1/3(w0)
  Mux1/1 -> xCoM pars/1
  one2/1 -> Gain/1
  Constant2/1 -> Gain1/1
  Demux/3 -> xCoM Pred Rel1/1(x)
  Demux1/3 -> xCoM Pred Rel1/2(v)
  Demux/1 -> xCoM Pred Rel/1(x)
  Demux1/1 -> xCoM Pred Rel/2(v)
  Demux/2 -> Terminator/1
  Demux1/2 -> Terminator1/1

== system Control_model_10DOF_fin/Control/Single_Support/Right Swing // Left Stance/Martijn Step adjustement/xCoM pred/xCoM part ==

== system Control_model_10DOF_fin/Control/Finish_Swing_Phase/Left Swing // Right Stance/Martijn Step adjustement/xCoM pred/Left swing correction/Left Swing ==
  Action Port : ActionPort  InitializeStates=reset  ActionType=else
  Constant : Constant  Value=[1; -1]
  se_corr : Outport
  wires:
  Constant/1 -> se_corr/1

== system Control_model_10DOF_fin/Control/Finish_Swing_Phase/Left Swing // Right Stance/Martijn Step adjustement/xCoM pred/Left swing correction/Right Swing ==
  Action Port : ActionPort  InitializeStates=reset  ActionType=then
  Constant : Constant  Value=[1; 1]
  se_corr : Outport
  wires:
  Constant/1 -> se_corr/1

== system Control_model_10DOF_fin/Control/Finish_Swing_Phase/Left Swing // Right Stance/Martijn Step adjustement/xCoM pred/xCoM Pred wrt x_m/xCoM Pred Rel ==
  note: 3.5 equation
  x : Inport
  v : Inport  Port=2
  w0 : Inport  Port=3
  Xp : Inport  Port=4
  T-t0 : Inport  Port=5
  Divide1 : Product  Inputs=**
  Divide2 : Product  Inputs=**
  Divide3 : Product  Inputs=**/
  Sum : Sum  Inputs=+-
  Sum1 : Sum  Inputs=+++
  Trigonometric Function : Trigonometry  Operator=sinh
  Trigonometric Function1 : Trigonometry  Operator=cosh
  xCoM Pred : Outport
  wires:
  Sum1/1 -> xCoM Pred/1
  Divide3/1 -> Sum1/3
  Divide2/1 -> Sum1/2
  v/1 -> Divide3/2
  Trigonometric Function1/1 -> Divide3/1
  Trigonometric Function/1 -> Divide2/2
  Sum/1 -> Divide2/1
  Xp/1 -> Sum1/1, Sum/2
  x/1 -> Sum/1
  w0/1 -> Divide1/2, Divide3/3
  T-t0/1 -> Divide1/1
  Divide1/1 -> Trigonometric Function/1, Trigonometric Function1/1

== system Control_model_10DOF_fin/Control/Finish_Swing_Phase/Left Swing // Right Stance/Martijn Step adjustement/xCoM pred/xCoM Pred wrt x_m/xCoM Pred Rel1 ==
  x : Inport
  v : Inport  Port=2
  w0 : Inport  Port=3
  Xp : Inport  Port=4
  T-t0 : Inport  Port=5
  Divide1 : Product  Inputs=**
  Divide2 : Product  Inputs=**
  Divide3 : Product  Inputs=**/
  Sum : Sum  Inputs=+-
  Sum1 : Sum  Inputs=+++
  Trigonometric Function : Trigonometry  Operator=sinh
  Trigonometric Function1 : Trigonometry  Operator=cosh
  xCoM Pred : Outport
  wires:
  Divide1/1 -> Trigonometric Function1/1, Trigonometric Function/1
  T-t0/1 -> Divide1/1
  w0/1 -> Divide1/2, Divide3/3
  x/1 -> Sum/1
  Xp/1 -> Sum/2, Sum1/1
  Sum/1 -> Divide2/1
  Trigonometric Function/1 -> Divide2/2
  Trigonometric Function1/1 -> Divide3/1
  v/1 -> Divide3/2
  Divide2/1 -> Sum1/2
  Divide3/1 -> Sum1/3
  Sum1/1 -> xCoM Pred/1

== system Control_model_10DOF_fin/Control/Finish_Swing_Phase/Right Swing // Left Stance1/Martijn Step adjustement/xCoM pred/Left swing correction/Left Swing ==
  Action Port : ActionPort  InitializeStates=reset  ActionType=else
  Constant : Constant  Value=[1; -1]
  se_corr : Outport
  wires:
  Constant/1 -> se_corr/1

== system Control_model_10DOF_fin/Control/Finish_Swing_Phase/Right Swing // Left Stance1/Martijn Step adjustement/xCoM pred/Left swing correction/Right Swing ==
  Action Port : ActionPort  InitializeStates=reset  ActionType=then
  Constant : Constant  Value=[1; 1]
  se_corr : Outport
  wires:
  Constant/1 -> se_corr/1

== system Control_model_10DOF_fin/Control/Finish_Swing_Phase/Right Swing // Left Stance1/Martijn Step adjustement/xCoM pred/xCoM Pred wrt x_m/xCoM Pred Rel ==
  note: 3.5 equation
  x : Inport
  v : Inport  Port=2
  w0 : Inport  Port=3
  Xp : Inport  Port=4
  T-t0 : Inport  Port=5
  Divide1 : Product  Inputs=**
  Divide2 : Product  Inputs=**
  Divide3 : Product  Inputs=**/
  Sum : Sum  Inputs=+-
  Sum1 : Sum  Inputs=+++
  Trigonometric Function : Trigonometry  Operator=sinh
  Trigonometric Function1 : Trigonometry  Operator=cosh
  xCoM Pred : Outport
  wires:
  Sum1/1 -> xCoM Pred/1
  Divide3/1 -> Sum1/3
  Divide2/1 -> Sum1/2
  v/1 -> Divide3/2
  Trigonometric Function1/1 -> Divide3/1
  Trigonometric Function/1 -> Divide2/2
  Sum/1 -> Divide2/1
  Xp/1 -> Sum1/1, Sum/2
  x/1 -> Sum/1
  w0/1 -> Divide1/2, Divide3/3
  T-t0/1 -> Divide1/1
  Divide1/1 -> Trigonometric Function/1, Trigonometric Function1/1

== system Control_model_10DOF_fin/Control/Finish_Swing_Phase/Right Swing // Left Stance1/Martijn Step adjustement/xCoM pred/xCoM Pred wrt x_m/xCoM Pred Rel1 ==
  x : Inport
  v : Inport  Port=2
  w0 : Inport  Port=3
  Xp : Inport  Port=4
  T-t0 : Inport  Port=5
  Divide1 : Product  Inputs=**
  Divide2 : Product  Inputs=**
  Divide3 : Product  Inputs=**/
  Sum : Sum  Inputs=+-
  Sum1 : Sum  Inputs=+++
  Trigonometric Function : Trigonometry  Operator=sinh
  Trigonometric Function1 : Trigonometry  Operator=cosh
  xCoM Pred : Outport
  wires:
  Divide1/1 -> Trigonometric Function1/1, Trigonometric Function/1
  T-t0/1 -> Divide1/1
  w0/1 -> Divide1/2, Divide3/3
  x/1 -> Sum/1
  Xp/1 -> Sum/2, Sum1/1
  Sum/1 -> Divide2/1
  Trigonometric Function/1 -> Divide2/2
  Trigonometric Function1/1 -> Divide3/1
  v/1 -> Divide3/2
  Divide2/1 -> Sum1/2
  Divide3/1 -> Sum1/3
  Sum1/1 -> xCoM Pred/1

== system Control_model_10DOF_fin/Control/Single_Support/Left Swing // Right Stance/Martijn Step adjustement/xCoM pred/Left swing correction/Left Swing ==
  Action Port : ActionPort  InitializeStates=reset  ActionType=else
  Constant : Constant  Value=[1; -1]
  se_corr : Outport
  wires:
  Constant/1 -> se_corr/1

== system Control_model_10DOF_fin/Control/Single_Support/Left Swing // Right Stance/Martijn Step adjustement/xCoM pred/Left swing correction/Right Swing ==
  Action Port : ActionPort  InitializeStates=reset  ActionType=then
  Constant : Constant  Value=[1; 1]
  se_corr : Outport
  wires:
  Constant/1 -> se_corr/1

== system Control_model_10DOF_fin/Control/Single_Support/Left Swing // Right Stance/Martijn Step adjustement/xCoM pred/xCoM Pred wrt x_m/xCoM Pred Rel ==
  note: 3.5 equation
  x : Inport
  v : Inport  Port=2
  w0 : Inport  Port=3
  Xp : Inport  Port=4
  T-t0 : Inport  Port=5
  Divide1 : Product  Inputs=**
  Divide2 : Product  Inputs=**
  Divide3 : Product  Inputs=**/
  Sum : Sum  Inputs=+-
  Sum1 : Sum  Inputs=+++
  Trigonometric Function : Trigonometry  Operator=sinh
  Trigonometric Function1 : Trigonometry  Operator=cosh
  xCoM Pred : Outport
  wires:
  Sum1/1 -> xCoM Pred/1
  Divide3/1 -> Sum1/3
  Divide2/1 -> Sum1/2
  v/1 -> Divide3/2
  Trigonometric Function1/1 -> Divide3/1
  Trigonometric Function/1 -> Divide2/2
  Sum/1 -> Divide2/1
  Xp/1 -> Sum1/1, Sum/2
  x/1 -> Sum/1
  w0/1 -> Divide1/2, Divide3/3
  T-t0/1 -> Divide1/1
  Divide1/1 -> Trigonometric Function/1, Trigonometric Function1/1

== system Control_model_10DOF_fin/Control/Single_Support/Left Swing // Right Stance/Martijn Step adjustement/xCoM pred/xCoM Pred wrt x_m/xCoM Pred Rel1 ==
  x : Inport
  v : Inport  Port=2
  w0 : Inport  Port=3
  Xp : Inport  Port=4
  T-t0 : Inport  Port=5
  Divide1 : Product  Inputs=**
  Divide2 : Product  Inputs=**
  Divide3 : Product  Inputs=**/
  Sum : Sum  Inputs=+-
  Sum1 : Sum  Inputs=+++
  Trigonometric Function : Trigonometry  Operator=sinh
  Trigonometric Function1 : Trigonometry  Operator=cosh
  xCoM Pred : Outport
  wires:
  Divide1/1 -> Trigonometric Function1/1, Trigonometric Function/1
  T-t0/1 -> Divide1/1
  w0/1 -> Divide1/2, Divide3/3
  x/1 -> Sum/1
  Xp/1 -> Sum/2, Sum1/1
  Sum/1 -> Divide2/1
  Trigonometric Function/1 -> Divide2/2
  Trigonometric Function1/1 -> Divide3/1
  v/1 -> Divide3/2
  Divide2/1 -> Sum1/2
  Divide3/1 -> Sum1/3
  Sum1/1 -> xCoM Pred/1

== system Control_model_10DOF_fin/Control/Single_Support/Right Swing // Left Stance/Martijn Step adjustement/xCoM pred/Left swing correction/Left Swing ==
  Action Port : ActionPort  InitializeStates=reset  ActionType=else
  Constant : Constant  Value=[1; -1]
  se_corr : Outport
  wires:
  Constant/1 -> se_corr/1

== system Control_model_10DOF_fin/Control/Single_Support/Right Swing // Left Stance/Martijn Step adjustement/xCoM pred/Left swing correction/Right Swing ==
  Action Port : ActionPort  InitializeStates=reset  ActionType=then
  Constant : Constant  Value=[1; 1]
  se_corr : Outport
  wires:
  Constant/1 -> se_corr/1

== system Control_model_10DOF_fin/Control/Single_Support/Right Swing // Left Stance/Martijn Step adjustement/xCoM pred/xCoM Pred wrt x_m/xCoM Pred Rel ==
  note: 3.5 equation
  x : Inport
  v : Inport  Port=2
  w0 : Inport  Port=3
  Xp : Inport  Port=4
  T-t0 : Inport  Port=5
  Divide1 : Product  Inputs=**
  Divide2 : Product  Inputs=**
  Divide3 : Product  Inputs=**/
  Sum : Sum  Inputs=+-
  Sum1 : Sum  Inputs=+++
  Trigonometric Function : Trigonometry  Operator=sinh
  Trigonometric Function1 : Trigonometry  Operator=cosh
  xCoM Pred : Outport
  wires:
  Sum1/1 -> xCoM Pred/1
  Divide3/1 -> Sum1/3
  Divide2/1 -> Sum1/2
  v/1 -> Divide3/2
  Trigonometric Function1/1 -> Divide3/1
  Trigonometric Function/1 -> Divide2/2
  Sum/1 -> Divide2/1
  Xp/1 -> Sum1/1, Sum/2
  x/1 -> Sum/1
  w0/1 -> Divide1/2, Divide3/3
  T-t0/1 -> Divide1/1
  Divide1/1 -> Trigonometric Function/1, Trigonometric Function1/1

== system Control_model_10DOF_fin/Control/Single_Support/Right Swing // Left Stance/Martijn Step adjustement/xCoM pred/xCoM Pred wrt x_m/xCoM Pred Rel1 ==
  x : Inport
  v : Inport  Port=2
  w0 : Inport  Port=3
  Xp : Inport  Port=4
  T-t0 : Inport  Port=5
  Divide1 : Product  Inputs=**
  Divide2 : Product  Inputs=**
  Divide3 : Product  Inputs=**/
  Sum : Sum  Inputs=+-
  Sum1 : Sum  Inputs=+++
  Trigonometric Function : Trigonometry  Operator=sinh
  Trigonometric Function1 : Trigonometry  Operator=cosh
  xCoM Pred : Outport
  wires:
  Divide1/1 -> Trigonometric Function1/1, Trigonometric Function/1
  T-t0/1 -> Divide1/1
  w0/1 -> Divide1/2, Divide3/3
  x/1 -> Sum/1
  Xp/1 -> Sum/2, Sum1/1
  Sum/1 -> Divide2/1
  Trigonometric Function/1 -> Divide2/2
  Trigonometric Function1/1 -> Divide3/1
  v/1 -> Divide3/2
  Divide2/1 -> Sum1/2
  Divide3/1 -> Sum1/3
  Sum1/1 -> xCoM Pred/1

== matlab function Control_model_10DOF_fin/10DoF Walker SimMechanics Model/Ankle EI/MATLAB Function ==
  data: joint input; torque output; validity_AEI parameter
function torque = fcn(joint,validity_AEI)

k=1000;

min=validity_AEI(1,1);
max=validity_AEI(1,2);

if joint<=min
    torque=k*(min-joint);
elseif joint>=max
    torque=k*(max-joint);
else
    torque=0;
end

== matlab function Control_model_10DOF_fin/10DoF Walker SimMechanics Model/Ankle EI1/MATLAB Function ==
  data: joint input; torque output; validity_AEI parameter
function torque = fcn(joint,validity_AEI)

k=1000;

min=validity_AEI(2,1);
max=validity_AEI(2,2);

if joint<=min
    torque=k*(min-joint);
elseif joint>=max
    torque=k*(max-joint);
else
    torque=0;
end

== matlab function Control_model_10DOF_fin/10DoF Walker SimMechanics Model/Ankle FE/MATLAB Function ==
  data: joint input; velocity input; desired_torque input; torque output; validity_angle parameter
function torque = fcn(joint,velocity,desired_torque,validity_angle)

kp=900;
kv=0.008;

min=validity_angle(1,1);
max=validity_angle(1,2);

if joint<=min
    torque=kp*(min-joint)-kv*velocity;
    if torque<=0
        torque=desired_torque;
    end
elseif joint>=max
    torque=kp*(max-joint)-kv*velocity;
    if torque>=0
        torque=desired_torque;
    end
else
    torque=desired_torque;
end

== matlab function Control_model_10DOF_fin/10DoF Walker SimMechanics Model/Ankle FE1/MATLAB Function ==
  data: joint input; velocity input; desired_torque input; torque output; validity_angle parameter
function torque = fcn(joint,velocity,desired_torque,validity_angle)

kp=900;
kv=0.008;

min=validity_angle(8,1);
max=validity_angle(8,2);

if joint<=min
    torque=kp*(min-joint)-kv*velocity;
    if torque<=0
        torque=desired_torque;
    end
elseif joint>=max
    torque=kp*(max-joint)-kv*velocity;
    if torque>=0
        torque=desired_torque;
    end
else
    torque=desired_torque;
end

== matlab function Control_model_10DOF_fin/10DoF Walker SimMechanics Model/Foot/GRF1 Heel/MATLAB Function1 ==
  data: x input; dx input; y input; dy input; z input; Fx output; dz input; Fy output; k input; Fz output
function [Fx,Fy,Fz]= fcn(x,dx,y,dy,z,dz,k)
%#codegen
% k=[5*10^4 10^4 0 10^4 0];
% k=[5*10^4 10^4 0 0 0];
% k=[0 0 0 0 0];

kp = k(1);
kv = k(2);
kpt = k(3);
kvt = k(4);
mu = k(5);

persistent prevContact;

if y>0
    Fy = 0;
    Fxz = [0;0];
    prevContact = [];
else
    if isempty(prevContact)
        prevContact = [x;z];
    end
    Current = [x;z];
    
    Fy = -kp*y-kv*dy;
%     Fxz = -kpt*(Current-prevContact)-kvt*[dx;dz];
    Fxz = -kvt*[dx;dz];
end

if Fy<0;
    Fy = 0;
%     prevContact = [];
end

mu=1;
if norm(Fxz)>mu*norm(Fy)
    Fxz = Fxz/norm(Fxz)*mu*norm(Fy);
end

Fx = Fxz(1);
Fz = Fxz(2);

== matlab function Control_model_10DOF_fin/10DoF Walker SimMechanics Model/Foot/GRF1 Toe/MATLAB Function1 ==
  data: x input; dx input; y input; dy input; z input; Fx output; dz input; Fy output; k input; Fz output
function [Fx,Fy,Fz]= fcn(x,dx,y,dy,z,dz,k)
%#codegen
% k=[5*10^4 10^4 0 10^4 0];
%k=[5*10^4 10^4 0 0 0];
% k=[0 0 0 0 0];

kp = k(1);
kv = k(2);
kpt = k(3);
kvt = k(4);
mu = k(5);

persistent prevContact;

if y>0
    Fy = 0;
    Fxz = [0;0];
    prevContact = [];
else
    if isempty(prevContact)
        prevContact = [x;z];
    end
    Current = [x;z];
    
    Fy = -kp*y-kv*dy;
%     Fxz = -kpt*(Current-prevContact)-kvt*[dx;dz];
    Fxz = -kvt*[dx;dz];
end

if Fy<0
    Fy = 0;
%     prevContact = [];
end

mu=1;
if norm(Fxz)>mu*norm(Fy)
    Fxz = Fxz/norm(Fxz)*mu*norm(Fy);
end

Fx = Fxz(1);
Fz = Fxz(2);

== matlab function Control_model_10DOF_fin/10DoF Walker SimMechanics Model/Foot/GRF2 Heel/MATLAB Function1 ==
  data: x input; dx input; y input; dy input; z input; Fx output; dz input; Fy output; k input; Fz output
 function [Fx,Fy,Fz]= fcn(x,dx,y,dy,z,dz,k)
%#codegen
% k=[5*10^4 10^4 0 10^4 0];
% k=[5*10^4 10^4 0 0 0];
% k=[0 0 0 0 0];

kp = k(1);
kv = k(2);
kpt = k(3);
kvt = k(4);
mu = k(5);

persistent prevContact;

if y>0
    Fy = 0;
    Fxz = [0;0];
    prevContact = [];
else
    if isempty(prevContact)
        prevContact = [x;z];
    end
    Current = [x;z];
    
    Fy = -kp*y-kv*dy;
%     Fxz = -kpt*(Current-prevContact)-kvt*[dx;dz];
    Fxz = -kvt*[dx;dz];
end

if Fy<0;
    Fy = 0;
%     prevContact = [];
end

mu=1;
if norm(Fxz)>mu*norm(Fy)
    Fxz = Fxz/norm(Fxz)*mu*norm(Fy);
end

Fx = Fxz(1);
Fz = Fxz(2);
